simulink model "torqueBalancingPHRIStandup_2016b"  (Simulink 8.8)
settings: Solver=FixedStepDiscrete  StartTime=0.0  StopTime="Config.SIMULATION_TIME "  FixedStep=Config.Ts  RelTol=1e-3  EnableMultiTasking=on
InitFcn:
  | cd(fileparts(which(bdroot)));
  | initTorqueBalancingPHRIStandup;
StopFcn:
  | cd(fileparts(which(bdroot)));
  | stopTorqueBalancingPHRIStandup;
undefined symbols (not defined in the file or in its folder): bVectorConstraintsFeet, bVectorConstraintsLegs, Config, ConstraintsMatrixFeet, ConstraintsMatrixLegs, Gain, HUMAN_DOF_FOR_SIMULINK, Reg, ROBOT_DOF, ROBOT_DOF_FOR_SIMULINK, Sat, Sm
libraries: WBToolboxLibrary x153, simulink x4
(part 3 of 3)

== system torqueBalancingPHRIStandup_2016b/Robot system/controller_QP/Compute joint torques/QPSolver ==
  LEFT_RIGHT_FOOT_IN_CONTACT : Inport
  HessianMatrixQP1Foot : Inport  Port=2
  gradientQP1Foot : Inport  Port=3
  ConstraintsMatrixQP1Foot : Inport  Port=4
  bVectorConstraintsQP1Foot : Inport  Port=5
  HessianMatrixQP2Feet : Inport  Port=6
  gradientQP2Feet : Inport  Port=7
  ConstraintsMatrixQP2Feet : Inport  Port=8
  bVectorConstraintsQp2Feet : Inport  Port=9
  state : Inport  Port=10
  Constant1 : Constant  Value=Config.USE_QP_SOLVER
  Level-2 MATLAB S-Function : M-S-Function  FunctionName=QPBalancingStandup
  Logical Operator1 : Logic  Operator=OR  AllPortsSameDT=off  OutDataTypeStr=boolean
  ON_GAZEBO 3 : Constant  Value=Config.SCOPES_ALL
  ON_GAZEBO 4 : Constant  Value=Config.SCOPES_QP
  Visualize eventual QP failures : Subsystem
  f0OneFoot : Outport
  f0TwoFeet : Outport  Port=2
  wires:
  Level-2 MATLAB S-Function/1 -> f0TwoFeet/1
  Level-2 MATLAB S-Function/2 -> Visualize eventual QP failures/1(exitFlagQP)  "Exit flag QP two feet"
  HessianMatrixQP1Foot/1 -> Level-2 MATLAB S-Function/7
  gradientQP1Foot/1 -> Level-2 MATLAB S-Function/8
  ConstraintsMatrixQP1Foot/1 -> Level-2 MATLAB S-Function/9
  bVectorConstraintsQP1Foot/1 -> Level-2 MATLAB S-Function/10
  Level-2 MATLAB S-Function/3 -> f0OneFoot/1
  Logical Operator1/1 -> Visualize eventual QP failures/Enable
  state/1 -> Visualize eventual QP failures/2(state)
  LEFT_RIGHT_FOOT_IN_CONTACT/1 -> Level-2 MATLAB S-Function/1
  HessianMatrixQP2Feet/1 -> Level-2 MATLAB S-Function/2
  gradientQP2Feet/1 -> Level-2 MATLAB S-Function/3
  ConstraintsMatrixQP2Feet/1 -> Level-2 MATLAB S-Function/4
  bVectorConstraintsQp2Feet/1 -> Level-2 MATLAB S-Function/5
  Constant1/1 -> Level-2 MATLAB S-Function/6
  ON_GAZEBO 3/1 -> Logical Operator1/1
  ON_GAZEBO 4/1 -> Logical Operator1/2

== system torqueBalancingPHRIStandup_2016b/Human system/Dump and visualize/Human data/Using Human Model/human joint data ==
  human_jointData : Inport
  Scope : Scope  NumInputPorts=6
  head : Selector  InputPortWidth=66  IndexOptions=Index vector (dialog)  Indices=[16 17 18]  OutputSizes=1
  jointData : Scope  NumInputPorts=16
  left_ankle : Selector  InputPortWidth=66  IndexOptions=Index vector (dialog)  Indices=[61 62 63]  OutputSizes=1
  left_ball_foot : Selector  InputPortWidth=66  IndexOptions=Index vector (dialog)  Indices=[64 65 66]  OutputSizes=1
  left_elbow : Selector  InputPortWidth=66  IndexOptions=Index vector (dialog)  Indices=[37 38 39]  OutputSizes=1
  left_hip : Selector  InputPortWidth=66  IndexOptions=Index vector (dialog)  Indices=[55 56 57]  OutputSizes=1
  left_knee : Selector  InputPortWidth=66  IndexOptions=Index vector (dialog)  Indices=[58 59 60]  OutputSizes=1
  left_shoulder : Selector  InputPortWidth=66  IndexOptions=Index vector (dialog)  Indices=[34 35 36]  OutputSizes=1
  left_shoulder_internal : Selector  InputPortWidth=66  IndexOptions=Index vector (dialog)  Indices=[31 32 33]  OutputSizes=1
  left_wrist : Selector  InputPortWidth=66  IndexOptions=Index vector (dialog)  Indices=[40 41 42]  OutputSizes=1
  neck : Selector  InputPortWidth=66  IndexOptions=Index vector (dialog)  Indices=[13 14 15]  OutputSizes=1
  right_ankle : Selector  InputPortWidth=66  IndexOptions=Index vector (dialog)  Indices=[49 50 51]  OutputSizes=1
  right_ball_foot : Selector  InputPortWidth=66  IndexOptions=Index vector (dialog)  Indices=[52 53 54]  OutputSizes=1
  right_elbow : Selector  InputPortWidth=66  IndexOptions=Index vector (dialog)  Indices=[25 26 27]  OutputSizes=1
  right_hip : Selector  InputPortWidth=66  IndexOptions=Index vector (dialog)  Indices=[43 44 45]  OutputSizes=1
  right_knee : Selector  InputPortWidth=66  IndexOptions=Index vector (dialog)  Indices=[46 47 48]  OutputSizes=1
  right_shoulder : Selector  InputPortWidth=66  IndexOptions=Index vector (dialog)  Indices=[22 23 24]  OutputSizes=1
  right_shoulder_internal : Selector  InputPortWidth=66  IndexOptions=Index vector (dialog)  Indices=[19 20 21]  OutputSizes=1
  right_wrist : Selector  InputPortWidth=66  IndexOptions=Index vector (dialog)  Indices=[28 29 30]  OutputSizes=1
  torso_1 : Selector  InputPortWidth=66  IndexOptions=Index vector (dialog)  Indices=[10 11 12]  OutputSizes=1
  torso_2 : Selector  InputPortWidth=66  IndexOptions=Index vector (dialog)  Indices=[7 8 9]  OutputSizes=1
  torso_3 : Selector  InputPortWidth=66  IndexOptions=Index vector (dialog)  Indices=[4 5 6]  OutputSizes=1
  torso_4 : Selector  InputPortWidth=66  IndexOptions=Index vector (dialog)  Indices=[1 2 3]  OutputSizes=1
  wires:
  torso_1/1 -> jointData/1
  torso_4/1 -> jointData/4
  torso_3/1 -> jointData/3
  torso_2/1 -> jointData/2
  right_shoulder_internal/1 -> jointData/6
  left_shoulder_internal/1 -> jointData/5
  left_hip/1 -> jointData/7
  right_hip/1 -> jointData/8
  left_shoulder/1 -> jointData/9
  right_shoulder/1 -> jointData/10
  left_knee/1 -> jointData/11
  right_knee/1 -> jointData/12
  left_elbow/1 -> jointData/13
  right_elbow/1 -> jointData/14
  left_ankle/1 -> jointData/15
  right_ankle/1 -> jointData/16
  human_jointData/1 -> head/1, left_ball_foot/1, left_wrist/1, neck/1, right_ball_foot/1, right_wrist/1, left_shoulder/1, right_hip/1, left_hip/1, right_shoulder_internal/1, torso_1/1, torso_2/1, torso_3/1, torso_4/1, left_shoulder_internal/1, right_shoulder/1, left_knee/1, right_knee/1, left_elbow/1, right_elbow/1, right_ankle/1, left_ankle/1
  head/1 -> Scope/1
  left_ball_foot/1 -> Scope/2
  left_wrist/1 -> Scope/3
  neck/1 -> Scope/4
  right_ball_foot/1 -> Scope/5
  right_wrist/1 -> Scope/6

== system torqueBalancingPHRIStandup_2016b/Human system/Dump and visualize/Human data/Using Human Model/human joint torques data ==
  human_jointTorquesData : Inport
  Scope : Scope  NumInputPorts=6
  head : Selector  InputPortWidth=66  IndexOptions=Index vector (dialog)  Indices=[16 17 18]  OutputSizes=1
  jointTorquesData : Scope  NumInputPorts=16
  left_ankle : Selector  InputPortWidth=66  IndexOptions=Index vector (dialog)  Indices=[61 62 63]  OutputSizes=1
  left_ball_foot : Selector  InputPortWidth=66  IndexOptions=Index vector (dialog)  Indices=[64 65 66]  OutputSizes=1
  left_elbow : Selector  InputPortWidth=66  IndexOptions=Index vector (dialog)  Indices=[37 38 39]  OutputSizes=1
  left_hip : Selector  InputPortWidth=66  IndexOptions=Index vector (dialog)  Indices=[55 56 57]  OutputSizes=1
  left_knee : Selector  InputPortWidth=66  IndexOptions=Index vector (dialog)  Indices=[58 59 60]  OutputSizes=1
  left_shoulder : Selector  InputPortWidth=66  IndexOptions=Index vector (dialog)  Indices=[34 35 36]  OutputSizes=1
  left_shoulder_internal : Selector  InputPortWidth=66  IndexOptions=Index vector (dialog)  Indices=[31 32 33]  OutputSizes=1
  left_wrist : Selector  InputPortWidth=66  IndexOptions=Index vector (dialog)  Indices=[40 41 42]  OutputSizes=1
  neck : Selector  InputPortWidth=66  IndexOptions=Index vector (dialog)  Indices=[13 14 15]  OutputSizes=1
  right_ankle : Selector  InputPortWidth=66  IndexOptions=Index vector (dialog)  Indices=[49 50 51]  OutputSizes=1
  right_ball_foot : Selector  InputPortWidth=66  IndexOptions=Index vector (dialog)  Indices=[52 53 54]  OutputSizes=1
  right_elbow : Selector  InputPortWidth=66  IndexOptions=Index vector (dialog)  Indices=[25 26 27]  OutputSizes=1
  right_hip : Selector  InputPortWidth=66  IndexOptions=Index vector (dialog)  Indices=[43 44 45]  OutputSizes=1
  right_knee : Selector  InputPortWidth=66  IndexOptions=Index vector (dialog)  Indices=[46 47 48]  OutputSizes=1
  right_shoulder : Selector  InputPortWidth=66  IndexOptions=Index vector (dialog)  Indices=[22 23 24]  OutputSizes=1
  right_shoulder_internal : Selector  InputPortWidth=66  IndexOptions=Index vector (dialog)  Indices=[19 20 21]  OutputSizes=1
  right_wrist : Selector  InputPortWidth=66  IndexOptions=Index vector (dialog)  Indices=[28 29 30]  OutputSizes=1
  torso_1 : Selector  InputPortWidth=66  IndexOptions=Index vector (dialog)  Indices=[10 11 12]  OutputSizes=1
  torso_2 : Selector  InputPortWidth=66  IndexOptions=Index vector (dialog)  Indices=[7 8 9]  OutputSizes=1
  torso_3 : Selector  InputPortWidth=66  IndexOptions=Index vector (dialog)  Indices=[4 5 6]  OutputSizes=1
  torso_4 : Selector  InputPortWidth=66  IndexOptions=Index vector (dialog)  Indices=[1 2 3]  OutputSizes=1
  wires:
  torso_1/1 -> jointTorquesData/1
  torso_4/1 -> jointTorquesData/4
  torso_3/1 -> jointTorquesData/3
  torso_2/1 -> jointTorquesData/2
  right_shoulder_internal/1 -> jointTorquesData/6
  left_shoulder_internal/1 -> jointTorquesData/5
  left_hip/1 -> jointTorquesData/7
  right_hip/1 -> jointTorquesData/8
  left_shoulder/1 -> jointTorquesData/9
  right_shoulder/1 -> jointTorquesData/10
  left_knee/1 -> jointTorquesData/11
  right_knee/1 -> jointTorquesData/12
  left_elbow/1 -> jointTorquesData/13
  right_elbow/1 -> jointTorquesData/14
  left_ankle/1 -> jointTorquesData/15
  right_ankle/1 -> jointTorquesData/16
  human_jointTorquesData/1 -> head/1, left_ball_foot/1, left_wrist/1, neck/1, right_ball_foot/1, right_wrist/1, left_shoulder/1, right_hip/1, left_hip/1, right_shoulder_internal/1, torso_1/1, torso_2/1, torso_3/1, torso_4/1, left_shoulder_internal/1, right_shoulder/1, left_knee/1, right_knee/1, left_elbow/1, right_elbow/1, right_ankle/1, left_ankle/1
  head/1 -> Scope/1
  left_ball_foot/1 -> Scope/2
  left_wrist/1 -> Scope/3
  neck/1 -> Scope/4
  right_ball_foot/1 -> Scope/5
  right_wrist/1 -> Scope/6

== system torqueBalancingPHRIStandup_2016b/Human system/Dump and visualize/Human data/Using Human Model/human joint velocities data ==
  human_jointVelocitiesData : Inport
  Scope : Scope  NumInputPorts=6
  head : Selector  InputPortWidth=66  IndexOptions=Index vector (dialog)  Indices=[16 17 18]  OutputSizes=1
  jointVelocitiesData : Scope  NumInputPorts=16
  left_ankle : Selector  InputPortWidth=66  IndexOptions=Index vector (dialog)  Indices=[61 62 63]  OutputSizes=1
  left_ball_foot : Selector  InputPortWidth=66  IndexOptions=Index vector (dialog)  Indices=[64 65 66]  OutputSizes=1
  left_elbow : Selector  InputPortWidth=66  IndexOptions=Index vector (dialog)  Indices=[37 38 39]  OutputSizes=1
  left_hip : Selector  InputPortWidth=66  IndexOptions=Index vector (dialog)  Indices=[55 56 57]  OutputSizes=1
  left_knee : Selector  InputPortWidth=66  IndexOptions=Index vector (dialog)  Indices=[58 59 60]  OutputSizes=1
  left_shoulder : Selector  InputPortWidth=66  IndexOptions=Index vector (dialog)  Indices=[34 35 36]  OutputSizes=1
  left_shoulder_internal : Selector  InputPortWidth=66  IndexOptions=Index vector (dialog)  Indices=[31 32 33]  OutputSizes=1
  left_wrist : Selector  InputPortWidth=66  IndexOptions=Index vector (dialog)  Indices=[40 41 42]  OutputSizes=1
  neck : Selector  InputPortWidth=66  IndexOptions=Index vector (dialog)  Indices=[13 14 15]  OutputSizes=1
  right_ankle : Selector  InputPortWidth=66  IndexOptions=Index vector (dialog)  Indices=[49 50 51]  OutputSizes=1
  right_ball_foot : Selector  InputPortWidth=66  IndexOptions=Index vector (dialog)  Indices=[52 53 54]  OutputSizes=1
  right_elbow : Selector  InputPortWidth=66  IndexOptions=Index vector (dialog)  Indices=[25 26 27]  OutputSizes=1
  right_hip : Selector  InputPortWidth=66  IndexOptions=Index vector (dialog)  Indices=[43 44 45]  OutputSizes=1
  right_knee : Selector  InputPortWidth=66  IndexOptions=Index vector (dialog)  Indices=[46 47 48]  OutputSizes=1
  right_shoulder : Selector  InputPortWidth=66  IndexOptions=Index vector (dialog)  Indices=[22 23 24]  OutputSizes=1
  right_shoulder_internal : Selector  InputPortWidth=66  IndexOptions=Index vector (dialog)  Indices=[19 20 21]  OutputSizes=1
  right_wrist : Selector  InputPortWidth=66  IndexOptions=Index vector (dialog)  Indices=[28 29 30]  OutputSizes=1
  torso_1 : Selector  InputPortWidth=66  IndexOptions=Index vector (dialog)  Indices=[10 11 12]  OutputSizes=1
  torso_2 : Selector  InputPortWidth=66  IndexOptions=Index vector (dialog)  Indices=[7 8 9]  OutputSizes=1
  torso_3 : Selector  InputPortWidth=66  IndexOptions=Index vector (dialog)  Indices=[4 5 6]  OutputSizes=1
  torso_4 : Selector  InputPortWidth=66  IndexOptions=Index vector (dialog)  Indices=[1 2 3]  OutputSizes=1
  wires:
  torso_1/1 -> jointVelocitiesData/1
  torso_4/1 -> jointVelocitiesData/4
  torso_3/1 -> jointVelocitiesData/3
  torso_2/1 -> jointVelocitiesData/2
  right_shoulder_internal/1 -> jointVelocitiesData/6
  left_shoulder_internal/1 -> jointVelocitiesData/5
  left_hip/1 -> jointVelocitiesData/7
  right_hip/1 -> jointVelocitiesData/8
  left_shoulder/1 -> jointVelocitiesData/9
  right_shoulder/1 -> jointVelocitiesData/10
  left_knee/1 -> jointVelocitiesData/11
  right_knee/1 -> jointVelocitiesData/12
  left_elbow/1 -> jointVelocitiesData/13
  right_elbow/1 -> jointVelocitiesData/14
  left_ankle/1 -> jointVelocitiesData/15
  right_ankle/1 -> jointVelocitiesData/16
  human_jointVelocitiesData/1 -> head/1, left_ball_foot/1, left_wrist/1, neck/1, right_ball_foot/1, right_wrist/1, left_shoulder/1, right_hip/1, left_hip/1, right_shoulder_internal/1, torso_1/1, torso_2/1, torso_3/1, torso_4/1, left_shoulder_internal/1, right_shoulder/1, left_knee/1, right_knee/1, left_elbow/1, right_elbow/1, right_ankle/1, left_ankle/1
  head/1 -> Scope/1
  left_ball_foot/1 -> Scope/2
  left_wrist/1 -> Scope/3
  neck/1 -> Scope/4
  right_ball_foot/1 -> Scope/5
  right_wrist/1 -> Scope/6

== system torqueBalancingPHRIStandup_2016b/Robot system/Robot State and References/Internal Coordinator/Base to fixed_link/LFoot to base link transform  ==
  qj : Inport
  inertial : Inport  Port=2
  w_H_link : Inport  Port=3
  w_H_base_fixed : Inport  Port=4
  Fixed base to imu transform : WBToolboxLibrary/wholeBodyModel/Kinematics/Forward Kinematics  frameName=Frames.IMU
  Fixed base to root link transform : WBToolboxLibrary/wholeBodyModel/Kinematics/Forward Kinematics  frameName=Frames.BASE
  Inv\* : Product  Inputs=/*  Multiplication=Matrix(*)
  "Inv\\*  " : Product  Inputs=/*  Multiplication=Matrix(*)
  Neck Position : WBToolboxLibrary/Utilities/Yarp Read  portName=Ports.NECK_POS  signalSize=6  timeout=0.5  blocking=off  timestamp=off  autoconnect=on  errorOnConnection=off
  Switch6 : Switch  Criteria=u2 > Threshold
  USE_IMU4EST_BASE : Constant  Value=Config.USE_IMU4EST_BASE
  fromImuToHomogeousTransformFCN : MATLAB Function  TreatAsAtomicUnit=on
  holder 1 : WBToolboxLibrary/Utilities/holder 
  holder 2 : WBToolboxLibrary/Utilities/holder 
  neck transform : Subsystem
  link_H_b : Outport
  wires:
  Switch6/1 -> link_H_b/1
  "Inv\\*  "/1 -> Switch6/3, fromImuToHomogeousTransformFCN/3(link_H_base)  "link_H_root"
  USE_IMU4EST_BASE/1 -> Switch6/2
  Inv\*/1 -> fromImuToHomogeousTransformFCN/1(imu_H_link), holder 1/1  "imu_H_link"
  holder 2/1 -> fromImuToHomogeousTransformFCN/4(inertial_0)
  Fixed base to imu transform/1 -> Inv\*/1
  holder 1/1 -> fromImuToHomogeousTransformFCN/2(imu_H_link_0)
  qj/1 -> Fixed base to imu transform/2, Fixed base to root link transform/2
  fromImuToHomogeousTransformFCN/1(w_H_b) -> Switch6/1
  Fixed base to root link transform/1 -> "Inv\\*  "/2
  inertial/1 -> holder 2/1, fromImuToHomogeousTransformFCN/5(inertial)
  Neck Position/1 -> neck transform/1(neck port)
  neck transform/1(neck position) -> fromImuToHomogeousTransformFCN/6(neck_pos)
  w_H_link/1 -> "Inv\\*  "/1, Inv\*/2
  w_H_base_fixed/1 -> Fixed base to root link transform/1, Fixed base to imu transform/1

== system torqueBalancingPHRIStandup_2016b/Robot system/Robot State and References/Internal Coordinator/Compute State Velocity/Feet Jacobians ==
  qj : Inport
  w_H_b : Inport  Port=2
  Jacobian LFoot : WBToolboxLibrary/wholeBodyModel/Jacobians/Jacobian  frameName=Frames.LEFT_FOOT
  Jacobian RFoot : WBToolboxLibrary/wholeBodyModel/Jacobians/Jacobian  frameName=Frames.RIGHT_FOOT
  J_LFoot : Outport
  J_RFoot : Outport  Port=2
  wires:
  Jacobian LFoot/1 -> J_LFoot/1
  Jacobian RFoot/1 -> J_RFoot/1
  w_H_b/1 -> Jacobian RFoot/1, Jacobian LFoot/1
  qj/1 -> Jacobian LFoot/2, Jacobian RFoot/2

== system torqueBalancingPHRIStandup_2016b/Robot system/Robot State and References/State Machine Standup/Compute State Velocity/Fixed Links Jacobians ==
  "state " : Inport
  qj : Inport  Port=2
  w_H_b : Inport  Port=3
  " " : WBToolboxLibrary/wholeBodyModel/Jacobians/Jacobian  frameName=Frames.LEFT_LEG
  "  " : WBToolboxLibrary/wholeBodyModel/Jacobians/Jacobian  frameName=Frames.RIGHT_LEG
  "   " : WBToolboxLibrary/wholeBodyModel/Jacobians/Jacobian  frameName=Frames.RIGHT_FOOT
  "       " : WBToolboxLibrary/wholeBodyModel/Jacobians/Jacobian  frameName=Frames.LEFT_FOOT
  Constant : Constant  Value=Config.iCubStandUp
  Legs in Contact : MATLAB Function  TreatAsAtomicUnit=on
  Switch1 : Switch  Criteria=u2 > Threshold  Threshold=0.1
  Switch2 : Switch  Criteria=u2 > Threshold  Threshold=0.1
  J_LeftFixed : Outport
  J_RightFixed : Outport  Port=2
  wires:
  Switch2/1 -> J_RightFixed/1
  Legs in Contact/1(legsInContact) -> Switch2/2, Switch1/2
  " "/1 -> Switch1/1
  "       "/1 -> Switch1/3
  "   "/1 -> Switch2/3
  "  "/1 -> Switch2/1
  "state "/1 -> Legs in Contact/2(state)
  Constant/1 -> Legs in Contact/1(icubStandup)
  Switch1/1 -> J_LeftFixed/1
  qj/1 -> "   "/2, "  "/2, "       "/2, " "/2
  w_H_b/1 -> "   "/1, " "/1, "       "/1, "  "/1

== system torqueBalancingPHRIStandup_2016b/Robot system/Robot State and References/State Machine Standup/Compute base to fixed link transform/LFoot to base link transform  ==
  qj : Inport
  inertial : Inport  Port=2
  w_H_link : Inport  Port=3
  w_H_base_fixed : Inport  Port=4
  Fixed base to imu transform : WBToolboxLibrary/wholeBodyModel/Kinematics/Forward Kinematics  frameName=Frames.IMU
  Fixed base to root link transform : WBToolboxLibrary/wholeBodyModel/Kinematics/Forward Kinematics  frameName=Frames.BASE
  Inv\* : Product  Inputs=/*  Multiplication=Matrix(*)
  "Inv\\*  " : Product  Inputs=/*  Multiplication=Matrix(*)
  Neck Position : WBToolboxLibrary/Utilities/Yarp Read  portName=Ports.NECK_POS  signalSize=6  timeout=0.5  blocking=off  timestamp=off  autoconnect=on  errorOnConnection=off
  Switch6 : Switch  Criteria=u2 > Threshold
  USE_IMU4EST_BASE : Constant  Value=Config.USE_IMU4EST_BASE
  fromImuToHomogeousTransformFCN : MATLAB Function  TreatAsAtomicUnit=on
  holder 1 : WBToolboxLibrary/Utilities/holder 
  holder 2 : WBToolboxLibrary/Utilities/holder 
  neck transform : Subsystem
  link_H_b : Outport
  wires:
  Switch6/1 -> link_H_b/1
  "Inv\\*  "/1 -> Switch6/3, fromImuToHomogeousTransformFCN/3(link_H_base)  "link_H_root"
  USE_IMU4EST_BASE/1 -> Switch6/2
  Inv\*/1 -> fromImuToHomogeousTransformFCN/1(imu_H_link), holder 1/1  "imu_H_link"
  holder 2/1 -> fromImuToHomogeousTransformFCN/4(inertial_0)
  Fixed base to imu transform/1 -> Inv\*/1
  holder 1/1 -> fromImuToHomogeousTransformFCN/2(imu_H_link_0)
  qj/1 -> Fixed base to imu transform/2, Fixed base to root link transform/2
  fromImuToHomogeousTransformFCN/1(w_H_b) -> Switch6/1
  Fixed base to root link transform/1 -> "Inv\\*  "/2
  inertial/1 -> holder 2/1, fromImuToHomogeousTransformFCN/5(inertial)
  Neck Position/1 -> neck transform/1(neck port)
  neck transform/1(neck position) -> fromImuToHomogeousTransformFCN/6(neck_pos)
  w_H_link/1 -> "Inv\\*  "/1, Inv\*/2
  w_H_base_fixed/1 -> Fixed base to root link transform/1, Fixed base to imu transform/1

== system torqueBalancingPHRIStandup_2016b/Robot system/Robot State and References/State Machine Standup/Compute base to fixed link transform/LLeg to base link transform ==
  qj : Inport
  inertial : Inport  Port=2
  w_H_link : Inport  Port=3
  w_H_base_fixed : Inport  Port=4
  Fixed base to imu transform : WBToolboxLibrary/wholeBodyModel/Kinematics/Forward Kinematics  frameName=Frames.IMU
  Fixed base to root link transform : WBToolboxLibrary/wholeBodyModel/Kinematics/Forward Kinematics  frameName=Frames.BASE
  Inv\* : Product  Inputs=/*  Multiplication=Matrix(*)
  "Inv\\*  " : Product  Inputs=/*  Multiplication=Matrix(*)
  Neck Position : WBToolboxLibrary/Utilities/Yarp Read  portName=Ports.NECK_POS  signalSize=6  timeout=0.5  blocking=off  timestamp=off  autoconnect=on  errorOnConnection=off
  Switch6 : Switch  Criteria=u2 > Threshold
  USE_IMU4EST_BASE : Constant  Value=Config.USE_IMU4EST_BASE
  fromImuToHomogeousTransformFCN : MATLAB Function  TreatAsAtomicUnit=on
  holder 1 : WBToolboxLibrary/Utilities/holder 
  holder 2 : WBToolboxLibrary/Utilities/holder 
  neck transform : Subsystem
  link_H_b : Outport
  wires:
  Switch6/1 -> link_H_b/1
  "Inv\\*  "/1 -> Switch6/3, fromImuToHomogeousTransformFCN/3(link_H_base)  "link_H_root"
  USE_IMU4EST_BASE/1 -> Switch6/2
  Inv\*/1 -> fromImuToHomogeousTransformFCN/1(imu_H_link), holder 1/1  "imu_H_link"
  holder 2/1 -> fromImuToHomogeousTransformFCN/4(inertial_0)
  Fixed base to imu transform/1 -> Inv\*/1
  holder 1/1 -> fromImuToHomogeousTransformFCN/2(imu_H_link_0)
  qj/1 -> Fixed base to imu transform/2, Fixed base to root link transform/2
  fromImuToHomogeousTransformFCN/1(w_H_b) -> Switch6/1
  Fixed base to root link transform/1 -> "Inv\\*  "/2
  inertial/1 -> holder 2/1, fromImuToHomogeousTransformFCN/5(inertial)
  Neck Position/1 -> neck transform/1(neck port)
  neck transform/1(neck position) -> fromImuToHomogeousTransformFCN/6(neck_pos)
  w_H_link/1 -> "Inv\\*  "/1, Inv\*/2
  w_H_base_fixed/1 -> Fixed base to root link transform/1, Fixed base to imu transform/1

== system torqueBalancingPHRIStandup_2016b/Robot system/controller_QP/Compute angular momentum integral/Compute base to fixed link transform/LFoot to base link transform  ==
  qj : Inport
  inertial : Inport  Port=2
  w_H_link : Inport  Port=3
  w_H_base_fixed : Inport  Port=4
  Fixed base to imu transform : WBToolboxLibrary/wholeBodyModel/Kinematics/Forward Kinematics  frameName=Frames.IMU
  Fixed base to root link transform : WBToolboxLibrary/wholeBodyModel/Kinematics/Forward Kinematics  frameName=Frames.BASE
  Inv\* : Product  Inputs=/*  Multiplication=Matrix(*)
  "Inv\\*  " : Product  Inputs=/*  Multiplication=Matrix(*)
  Neck Position : WBToolboxLibrary/Utilities/Yarp Read  portName=Ports.NECK_POS  signalSize=6  timeout=0.5  blocking=off  timestamp=off  autoconnect=on  errorOnConnection=off
  Switch6 : Switch  Criteria=u2 > Threshold
  USE_IMU4EST_BASE : Constant  Value=Config.USE_IMU4EST_BASE
  fromImuToHomogeousTransformFCN : MATLAB Function  TreatAsAtomicUnit=on
  holder 1 : WBToolboxLibrary/Utilities/holder 
  holder 2 : WBToolboxLibrary/Utilities/holder 
  neck transform : Subsystem
  link_H_b : Outport
  wires:
  Switch6/1 -> link_H_b/1
  "Inv\\*  "/1 -> Switch6/3, fromImuToHomogeousTransformFCN/3(link_H_base)  "link_H_root"
  USE_IMU4EST_BASE/1 -> Switch6/2
  Inv\*/1 -> fromImuToHomogeousTransformFCN/1(imu_H_link), holder 1/1  "imu_H_link"
  holder 2/1 -> fromImuToHomogeousTransformFCN/4(inertial_0)
  Fixed base to imu transform/1 -> Inv\*/1
  holder 1/1 -> fromImuToHomogeousTransformFCN/2(imu_H_link_0)
  qj/1 -> Fixed base to imu transform/2, Fixed base to root link transform/2
  fromImuToHomogeousTransformFCN/1(w_H_b) -> Switch6/1
  Fixed base to root link transform/1 -> "Inv\\*  "/2
  inertial/1 -> holder 2/1, fromImuToHomogeousTransformFCN/5(inertial)
  Neck Position/1 -> neck transform/1(neck port)
  neck transform/1(neck position) -> fromImuToHomogeousTransformFCN/6(neck_pos)
  w_H_link/1 -> "Inv\\*  "/1, Inv\*/2
  w_H_base_fixed/1 -> Fixed base to root link transform/1, Fixed base to imu transform/1

== system torqueBalancingPHRIStandup_2016b/Robot system/controller_QP/Compute angular momentum integral/Compute base to fixed link transform/LLeg to base link transform ==
  qj : Inport
  inertial : Inport  Port=2
  w_H_link : Inport  Port=3
  w_H_base_fixed : Inport  Port=4
  Fixed base to imu transform : WBToolboxLibrary/wholeBodyModel/Kinematics/Forward Kinematics  frameName=Frames.IMU
  Fixed base to root link transform : WBToolboxLibrary/wholeBodyModel/Kinematics/Forward Kinematics  frameName=Frames.BASE
  Inv\* : Product  Inputs=/*  Multiplication=Matrix(*)
  "Inv\\*  " : Product  Inputs=/*  Multiplication=Matrix(*)
  Neck Position : WBToolboxLibrary/Utilities/Yarp Read  portName=Ports.NECK_POS  signalSize=6  timeout=0.5  blocking=off  timestamp=off  autoconnect=on  errorOnConnection=off
  Switch6 : Switch  Criteria=u2 > Threshold
  USE_IMU4EST_BASE : Constant  Value=Config.USE_IMU4EST_BASE
  fromImuToHomogeousTransformFCN : MATLAB Function  TreatAsAtomicUnit=on
  holder 1 : WBToolboxLibrary/Utilities/holder 
  holder 2 : WBToolboxLibrary/Utilities/holder 
  neck transform : Subsystem
  link_H_b : Outport
  wires:
  Switch6/1 -> link_H_b/1
  "Inv\\*  "/1 -> Switch6/3, fromImuToHomogeousTransformFCN/3(link_H_base)  "link_H_root"
  USE_IMU4EST_BASE/1 -> Switch6/2
  Inv\*/1 -> fromImuToHomogeousTransformFCN/1(imu_H_link), holder 1/1  "imu_H_link"
  holder 2/1 -> fromImuToHomogeousTransformFCN/4(inertial_0)
  Fixed base to imu transform/1 -> Inv\*/1
  holder 1/1 -> fromImuToHomogeousTransformFCN/2(imu_H_link_0)
  qj/1 -> Fixed base to imu transform/2, Fixed base to root link transform/2
  fromImuToHomogeousTransformFCN/1(w_H_b) -> Switch6/1
  Fixed base to root link transform/1 -> "Inv\\*  "/2
  inertial/1 -> holder 2/1, fromImuToHomogeousTransformFCN/5(inertial)
  Neck Position/1 -> neck transform/1(neck port)
  neck transform/1(neck position) -> fromImuToHomogeousTransformFCN/6(neck_pos)
  w_H_link/1 -> "Inv\\*  "/1, Inv\*/2
  w_H_base_fixed/1 -> Fixed base to root link transform/1, Fixed base to imu transform/1

== system torqueBalancingPHRIStandup_2016b/Robot system/controller_QP/Compute joint torques/QPSolver/Visualize eventual QP failures ==
  exitFlagQP : Inport
  state : Inport  Port=2
  Enable : EnablePort
  "QP status (0: no failure, 1: not using)" : Scope  NumInputPorts=2
  wires:
  exitFlagQP/1 -> "QP status (0: no failure, 1: not using)"/1  "exitFlagQP"
  state/1 -> "QP status (0: no failure, 1: not using)"/2

== system torqueBalancingPHRIStandup_2016b/Robot system/Robot State and References/Internal Coordinator/Base to fixed_link/LFoot to base link transform /neck transform ==
  neck port : Inport
  Constant : Constant  Value=zeros(3,1)
  Gain : Gain  Gain=pi/180
  Selector1 : Selector  InputPortWidth=6  IndexOptions=Index vector (dialog)  Indices=[1:3]  OutputSizes=1
  Switch : Switch  Criteria=u2 > Threshold
  USE_IMU4EST_BASE1 : Constant  Value=Config.CORRECT_NECK_IMU
  neck position : Outport
  wires:
  neck port/1 -> Gain/1
  USE_IMU4EST_BASE1/1 -> Switch/2
  Switch/1 -> neck position/1
  Gain/1 -> Selector1/1
  Constant/1 -> Switch/3
  Selector1/1 -> Switch/1  "neck pos"

== system torqueBalancingPHRIStandup_2016b/Robot system/Robot State and References/State Machine Standup/Compute base to fixed link transform/LFoot to base link transform /neck transform ==
  neck port : Inport
  Constant : Constant  Value=zeros(3,1)
  Gain : Gain  Gain=pi/180
  Selector1 : Selector  InputPortWidth=6  IndexOptions=Index vector (dialog)  Indices=[1:3]  OutputSizes=1
  Switch : Switch  Criteria=u2 > Threshold
  USE_IMU4EST_BASE1 : Constant  Value=Config.CORRECT_NECK_IMU
  neck position : Outport
  wires:
  neck port/1 -> Gain/1
  USE_IMU4EST_BASE1/1 -> Switch/2
  Switch/1 -> neck position/1
  Gain/1 -> Selector1/1
  Constant/1 -> Switch/3
  Selector1/1 -> Switch/1  "neck pos"

== system torqueBalancingPHRIStandup_2016b/Robot system/Robot State and References/State Machine Standup/Compute base to fixed link transform/LLeg to base link transform/neck transform ==
  neck port : Inport
  Constant : Constant  Value=zeros(3,1)
  Gain : Gain  Gain=pi/180
  Selector1 : Selector  InputPortWidth=6  IndexOptions=Index vector (dialog)  Indices=[1:3]  OutputSizes=1
  Switch : Switch  Criteria=u2 > Threshold
  USE_IMU4EST_BASE1 : Constant  Value=Config.CORRECT_NECK_IMU
  neck position : Outport
  wires:
  neck port/1 -> Gain/1
  USE_IMU4EST_BASE1/1 -> Switch/2
  Switch/1 -> neck position/1
  Gain/1 -> Selector1/1
  Constant/1 -> Switch/3
  Selector1/1 -> Switch/1  "neck pos"

== system torqueBalancingPHRIStandup_2016b/Robot system/controller_QP/Compute angular momentum integral/Compute base to fixed link transform/LFoot to base link transform /neck transform ==
  neck port : Inport
  Constant : Constant  Value=zeros(3,1)
  Gain : Gain  Gain=pi/180
  Selector1 : Selector  InputPortWidth=6  IndexOptions=Index vector (dialog)  Indices=[1:3]  OutputSizes=1
  Switch : Switch  Criteria=u2 > Threshold
  USE_IMU4EST_BASE1 : Constant  Value=Config.CORRECT_NECK_IMU
  neck position : Outport
  wires:
  neck port/1 -> Gain/1
  USE_IMU4EST_BASE1/1 -> Switch/2
  Switch/1 -> neck position/1
  Gain/1 -> Selector1/1
  Constant/1 -> Switch/3
  Selector1/1 -> Switch/1  "neck pos"

== system torqueBalancingPHRIStandup_2016b/Robot system/controller_QP/Compute angular momentum integral/Compute base to fixed link transform/LLeg to base link transform/neck transform ==
  neck port : Inport
  Constant : Constant  Value=zeros(3,1)
  Gain : Gain  Gain=pi/180
  Selector1 : Selector  InputPortWidth=6  IndexOptions=Index vector (dialog)  Indices=[1:3]  OutputSizes=1
  Switch : Switch  Criteria=u2 > Threshold
  USE_IMU4EST_BASE1 : Constant  Value=Config.CORRECT_NECK_IMU
  neck position : Outport
  wires:
  neck port/1 -> Gain/1
  USE_IMU4EST_BASE1/1 -> Switch/2
  Switch/1 -> neck position/1
  Gain/1 -> Selector1/1
  Constant/1 -> Switch/3
  Selector1/1 -> Switch/1  "neck pos"

== matlab function Robot system/controller_QP/Compute angular momentum integral/Compute base to fixed link transform/LFoot to base link transform /fromImuToHomogeousTransformFCN ==
  data: imu_H_link input double; imu_H_link_0 input double; link_H_base input double; inertial_0 input double; inertial input double; neck_pos input double; w_H_b output double; Config parameter double
function w_H_b = worldToBaseTransformWithIMUFCN(imu_H_link,imu_H_link_0,link_H_base,inertial_0,inertial,neck_pos,Config)

    w_H_b = worldToBaseTransformWithIMU(imu_H_link,imu_H_link_0,link_H_base,inertial_0,inertial,neck_pos,Config);

end

== matlab function Robot system/Robot State and References/Internal Coordinator/Base to fixed_link/LFoot to base link transform /fromImuToHomogeousTransformFCN ==
  data: imu_H_link input double; imu_H_link_0 input double; link_H_base input double; inertial_0 input double; inertial input double; neck_pos input double; w_H_b output double; Config parameter double
function w_H_b = worldToBaseTransformWithIMUFCN(imu_H_link,imu_H_link_0,link_H_base,inertial_0,inertial,neck_pos,Config)

    w_H_b = worldToBaseTransformWithIMU(imu_H_link,imu_H_link_0,link_H_base,inertial_0,inertial,neck_pos,Config);

end

== matlab function Robot system/Robot State and References/State Machine Standup/Compute base to fixed link transform/LLeg to base link transform/fromImuToHomogeousTransformFCN ==
  data: imu_H_link input double; imu_H_link_0 input double; link_H_base input double; inertial_0 input double; inertial input double; neck_pos input double; w_H_b output double; Config parameter double
function w_H_b = worldToBaseTransformWithIMUFCN(imu_H_link,imu_H_link_0,link_H_base,inertial_0,inertial,neck_pos,Config)

    w_H_b = worldToBaseTransformWithIMU(imu_H_link,imu_H_link_0,link_H_base,inertial_0,inertial,neck_pos,Config);

end

== matlab function Robot system/controller_QP/Compute angular momentum integral/Compute base to fixed link transform/LLeg to base link transform/fromImuToHomogeousTransformFCN ==
  data: imu_H_link input double; imu_H_link_0 input double; link_H_base input double; inertial_0 input double; inertial input double; neck_pos input double; w_H_b output double; Config parameter double
function w_H_b = worldToBaseTransformWithIMUFCN(imu_H_link,imu_H_link_0,link_H_base,inertial_0,inertial,neck_pos,Config)

    w_H_b = worldToBaseTransformWithIMU(imu_H_link,imu_H_link_0,link_H_base,inertial_0,inertial,neck_pos,Config);

end

== matlab function Robot system/Robot State and References/Internal Coordinator/Compute State Velocity/Compute Base Velocity ==
  data: J_LeftFoot input double; J_RightFoot input double; feetInContact input double; nu_b output double; qjDot input double; Reg parameter double
function nu_b = computeBaseVelocityFCN(J_LeftFoot, J_RightFoot, feetInContact, qjDot, Reg)

    nu_b = computeBaseVelocity(J_LeftFoot, J_RightFoot, feetInContact, qjDot, Reg);
end

== matlab function Robot system/Dynamics and Kinematics/Dynamics/Add motors reflected inertias/Add motor reflected inertias ==
  data: M input double; M_with_inertia output double; Config parameter double
function M_with_inertia = addMotorsInertiaFCN(M,Config)

    M_with_inertia = addMotorsInertia(M,Config);

end

== matlab function Robot system/Robot State and References/State Machine Standup/Compute State Velocity/Compute Base Velocity ==
  data: J_LeftFixedLink input double; J_RightFixedLink input double; feetInContact input double; nu_b output double; qjDot input double; Reg parameter double
function nu_b = computeBaseVelocityFCN(J_LeftFixedLink, J_RightFixedLink, feetInContact, qjDot, Reg)

    nu_b = computeBaseVelocity(J_LeftFixedLink, J_RightFixedLink, feetInContact, qjDot, Reg);
end

== matlab function Robot system/Robot State and References/State Machine Standup/Compute base to fixed link transform/LFoot to base link transform /fromImuToHomogeousTransformFCN ==
  data: imu_H_link input double; imu_H_link_0 input double; link_H_base input double; inertial_0 input double; inertial input double; neck_pos input double; w_H_b output double; Config parameter double
function w_H_b = worldToBaseTransformWithIMUFCN(imu_H_link,imu_H_link_0,link_H_base,inertial_0,inertial,neck_pos,Config)

    w_H_b = worldToBaseTransformWithIMU(imu_H_link,imu_H_link_0,link_H_base,inertial_0,inertial,neck_pos,Config);

end

== matlab function Robot system/Dynamics and Kinematics/Kinematics/Legs in Contact ==
  data: icubStandup input double; legsInContact output double; state input double
function legsInContact = legsContactDetectorFCN(icubStandup,state)

   legsInContact = legsContactDetector(icubStandup,state);
end

== matlab function Robot system/Robot State and References/Internal Coordinator/Reference Generator CoM ==
  data: pos_CoM_0 input double; t input double; references_CoM output double; Config parameter double
function references_CoM = referenceGeneratorCoMFCN(pos_CoM_0, t, Config)

    references_CoM = referenceGeneratorCoM(pos_CoM_0, t, Config);
end

== matlab function Robot system/controller_QP/Compute angular momentum integral/Legs in Contact ==
  data: icubStandup input double; legsInContact output double; state input double
function legsInContact = legsContactDetectorFCN(icubStandup,state)

   legsInContact = legsContactDetector(icubStandup,state);
end

== matlab function Robot system/controller_QP/Compute joint torques (motor reflected inertia)/(transpose(T*Gamma))^{-1}*I_m*(T*Gamma)^{-1} ==
  data: reflectedInertia output double; Config parameter double
function reflectedInertia  = computeMotorsInertiaFCN(Config)

    [reflectedInertia] = computeMotorsInertia(Config);

end

== matlab function Robot system/Robot State and References/State Machine Standup/stateMachineStandupFCN ==
  data: wrench_rightFoot input double; wrench_leftFoot input double; w_H_b output double; constraints output double; CoM_des output double; qj_des output double; wrench_leftHand input double; wrench_rightHand input double; xCoM_0 input double; qj_0 input double; xCoM input double; l_sole_H_b input double; l_upper_leg_contact_H_b input double; t input double; STANDUP_WITH_HUMAN_FORCE input double; MEASURED_FT input double; STANDUP_WITH_HUMAN_TORQUE input double; Sm parameter double; impedances output double; KPCoM output double; KDCoM output double; Gain parameter double; currentState output double; jointsAndCoMSmoothingTime output double; fArms_phri input double
function [w_H_b, constraints, CoM_des, qj_des, impedances, KPCoM, KDCoM, currentState, jointsAndCoMSmoothingTime] = ...
             stateMachineStandupFCN(wrench_rightFoot, wrench_leftFoot, wrench_leftHand, wrench_rightHand, xCoM_0, qj_0, xCoM, l_sole_H_b, l_upper_leg_contact_H_b, t, STANDUP_WITH_HUMAN_FORCE, MEASURED_FT, STANDUP_WITH_HUMAN_TORQUE, Sm, Gain, fArms_phri)
         
         [w_H_b, constraints, CoM_des, qj_des, impedances, KPCoM, KDCoM, currentState, jointsAndCoMSmoothingTime] = ...
             stateMachineStandup(wrench_rightFoot, wrench_leftFoot, wrench_leftHand, wrench_rightHand, xCoM_0, qj_0, xCoM, l_sole_H_b, l_upper_leg_contact_H_b, t, STANDUP_WITH_HUMAN_FORCE, MEASURED_FT, STANDUP_WITH_HUMAN_TORQUE, Sm, Gain, fArms_phri);
end

== matlab function Robot system/Robot State and References/State Machine Standup/Compute State Velocity/Fixed Links Jacobians/Legs in Contact ==
  data: icubStandup input double; legsInContact output double; state input double
function legsInContact = legsContactDetectorFCN(icubStandup,state)

   legsInContact = legsContactDetector(icubStandup,state);
end

== matlab function Robot system/robot world to human feet transformation/MATLAB Function ==
  data: w_H_humanLeftFeet output double; w_H_robotLeftFeet input double; w_H_robotRightFeet input double; w_H_humanRightFeet output double
function [w_H_humanLeftFeet, w_H_humanRightFeet ]= fcn(w_H_robotLeftFeet,w_H_robotRightFeet)

    %% Fixed transformation from the robot feet to human feet defined
    %  human-forces-provider module configuration
    robotLeftFeet_H_humanLeftFeet = [-1.0   0.0     0.0     0.59;
                                      0.0  -1.0     0.0    -0.2549;
                                      0.0   0.0     1.0     0.0;
                                      0.0   0.0     0.0     1.0];
                                  
    robotRightFeet_H_humanRightFeet = [-1.0   0.0     0.0     0.59;
                                        0.0  -1.0     0.0    -0.2549;
                                        0.0   0.0     1.0     0.0;
                                        0.0   0.0     0.0     1.0];
                                  
    w_H_humanLeftFeet  = w_H_robotLeftFeet * robotLeftFeet_H_humanLeftFeet;
    
    w_H_humanRightFeet = w_H_robotRightFeet * robotRightFeet_H_humanRightFeet;

end

== matlab function Human system/Robot Model Position Control/getJointRef ==
  data: sim_time input double; q input double; state input double; joint_ref output double
function joint_ref = getJointRef(sim_time, q, state)

    joint_ref        = q;
    joint_references = [-0.2973   -0.0000   -0.0000   -0.1376    0.1919   -0.0000    0.5629   -0.1376    0.1929   -0.0000    0.5629   -0.0003   -0.0001   -0.0001   -0.0008    0.0012    0.0001   -0.0004    0.0000    0.0001   -0.0008    0.0012   -0.0001;
                         0.1873    0.0000   -0.0000    0.1296    0.1901    0.0019    0.6084    0.1296    0.1901    0.0019    0.6084   -0.0007   -0.0001   -0.0001   -0.0017    0.0025    0.0001   -0.0007   -0.0000    0.0000   -0.0017    0.0025   -0.0001;
                         0.1873   -0.0000   -0.0000    0.1217    0.1896   -0.0004    1.1403    0.1217    0.1896   -0.0004    1.1403   -0.0014   -0.0001   -0.0000   -0.0023    0.0032    0.0000   -0.0014   -0.0000    0.0000   -0.0023    0.0032   -0.0000];

    if state < 4 && sim_time > 2
            
        joint_ref    = joint_references(state,:)';
        
    elseif state >= 4
        
        joint_ref    = joint_references(3,:)';
        
    end
              
end

== matlab function Robot system/controller_QP/Balancing Controller  ==
  data: tauModel output double; Sigma output double; NA output double; f_HDot output double; HessianMatrixQP1Foot output double; gradientQP1Foot output double; ConstraintsMatrixQP1Foot output double; bVectorConstraintsQp1Foot output double; HessianMatrixQP2FeetOrLegs output double; gradientQP2FeetOrLegs output double; ConstraintsMatrixQP2FeetOrLegs output double; bVectorConstraintsQp2FeetOrLegs output double; constraints input double; ROBOT_DOF_FOR_SIMULINK input double; HUMAN_DOF_FOR_SIMULINK input double; ConstraintsMatrix input double; bVectorConstraints input double; qj input double; qjDes input double; nu input double; M input double; h input double; L input double; intLw input double; w_H_l_contact input double; w_H_r_contact input double; JL input double; JR input double; dJL_nu input double; dJR_nu input double; xCoM input double; J_CoM input double; desired_x_dx_ddx_CoM input double; CMM input double; gainsPCOM input double; gainsDCOM input double; impedances input double; Reg parameter double; errorCoM output double; f_noQP output double; Gain parameter double; w_H_lArm input double; w_H_rArm input double; JLArm input double; JRArm input double; dJLArm_nu input double; dJRArm_nu input double; LArmWrench input double; RArmWrench input double; STANDUP_WITH_HUMAN_FORCE input double; MEASURED_FT input double; STANDUP_WITH_HUMAN_TORQUE input double; human_w_H_b input double; human_qj input double; human_nu_b input double; human_dqj input double; human_M input double; human_h input double; human_torques input double; human_w_H_l_contact input double; human_w_H_r_contact input double; human_JL input double; human_JR input double; human_dJL_nu input double; human_dJR_nu input double; human_w_H_lArm_contact input double; human_w_H_rArm_contact input double; human_JLArm input double; human_JRArm input double; human_dJLArm_nu input double; human_dJRArm_nu input double; correctionFromSupportForce output double; L_error output double; V output double; alpha output double; state input double; robot_torques input double; fArms output double; phri_human_feet_wrench output double; phri_robot_feet_wrench output double; correctionFromSupportTorque output double
function [tauModel, Sigma, NA, f_HDot, ...
          HessianMatrixQP1Foot, gradientQP1Foot, ConstraintsMatrixQP1Foot, bVectorConstraintsQp1Foot, ...
          HessianMatrixQP2FeetOrLegs, gradientQP2FeetOrLegs, ConstraintsMatrixQP2FeetOrLegs, bVectorConstraintsQp2FeetOrLegs, ...
          errorCoM, f_noQP, correctionFromSupportForce, L_error, V, alpha, fArms, phri_human_feet_wrench, phri_robot_feet_wrench, correctionFromSupportTorque] =  ...
              balancingControllerStandupFCN(constraints, ROBOT_DOF_FOR_SIMULINK, HUMAN_DOF_FOR_SIMULINK, ConstraintsMatrix, bVectorConstraints, ...
                                         qj, qjDes, nu, M, h, L, intLw, w_H_l_contact, w_H_r_contact, JL, JR, dJL_nu, dJR_nu, xCoM, J_CoM, desired_x_dx_ddx_CoM, CMM, ...
                                         gainsPCOM, gainsDCOM, impedances, Reg, Gain, w_H_lArm, w_H_rArm, JLArm, JRArm, dJLArm_nu, dJRArm_nu,...
                                         LArmWrench, RArmWrench, STANDUP_WITH_HUMAN_FORCE, MEASURED_FT, STANDUP_WITH_HUMAN_TORQUE, ...
                                         human_w_H_b, human_qj, human_nu_b, human_dqj, human_M, human_h, human_torques, ...
                                         human_w_H_l_contact, human_w_H_r_contact, human_JL, human_JR, human_dJL_nu, human_dJR_nu,...
                                         human_w_H_lArm_contact, human_w_H_rArm_contact, human_JLArm, human_JRArm, human_dJLArm_nu, human_dJRArm_nu,...
                                         state, robot_torques)
           
   [tauModel, Sigma, NA, f_HDot, ...
          HessianMatrixQP1Foot, gradientQP1Foot, ConstraintsMatrixQP1Foot, bVectorConstraintsQp1Foot, ...
          HessianMatrixQP2FeetOrLegs, gradientQP2FeetOrLegs, ConstraintsMatrixQP2FeetOrLegs, bVectorConstraintsQp2FeetOrLegs, ...
          errorCoM, f_noQP, correctionFromSupportForce, L_error, V, alpha, fArms, phri_human_feet_wrench, phri_robot_feet_wrench, correctionFromSupportTorque] =  ...
              balancingControllerStandup(constraints, ROBOT_DOF_FOR_SIMULINK, HUMAN_DOF_FOR_SIMULINK, ConstraintsMatrix, bVectorConstraints, ...
                                         qj, qjDes, nu, M, h, L, intLw, w_H_l_contact, w_H_r_contact, JL, JR, dJL_nu, dJR_nu, xCoM, J_CoM, desired_x_dx_ddx_CoM, CMM, ...
                                         gainsPCOM, gainsDCOM, impedances, Reg, Gain, w_H_lArm, w_H_rArm, JLArm, JRArm, dJLArm_nu, dJRArm_nu,...
                                         LArmWrench, RArmWrench, STANDUP_WITH_HUMAN_FORCE, MEASURED_FT, STANDUP_WITH_HUMAN_TORQUE, ...
                                         human_w_H_b, human_qj, human_nu_b, human_dqj, human_M, human_h, human_torques, ...
                                         human_w_H_l_contact, human_w_H_r_contact, human_JL, human_JR, human_dJL_nu, human_dJR_nu,...
                                         human_w_H_lArm_contact, human_w_H_rArm_contact, human_JLArm, human_JRArm, human_dJLArm_nu, human_dJRArm_nu,...
                                         state, robot_torques);
end

== matlab function Robot system/emergency stop: joint limits/MATLAB Function ==
  data: umin input double; umax input double; u input double; inRange output double; tol input double
function inRange = checkRangeFCN(umin, umax, u, tol)

    inRange = checkRange(umin, umax, u, tol);
end

== matlab function Robot system/controller_QP/Compute angular momentum integral/References for H ==
  data: qjErr input double; JL input double; JR input double; nu_b_equivalent output double; Reg parameter double; activeFeetConstraints input double
function nu_b_equivalent = generateReferencesForH_FCN(qjErr, JL, JR, Reg, activeFeetConstraints)

    if activeFeetConstraints(1) == 1
    
        pinvJb          = (JL(:,1:6)'*JL(:,1:6) + Reg.pinvDamp_nu_b*eye(6))\JL(:,1:6)';
        nu_b_equivalent = -pinvJb*JL(:,7:end)*qjErr;
    else
    
        pinvJb          = (JR(:,1:6)'*JR(:,1:6) + Reg.pinvDamp_nu_b*eye(6))\JR(:,1:6)';
        nu_b_equivalent = -pinvJb*JR(:,7:end)*qjErr;
    end
end

== matlab function Robot system/Robot State and References/State Machine Standup/Visualise extrnal wrenches/Compute current threshold ==
  data: thresholdContactLeftHand output double; thresholdContactRightHand output double; state input double; thresholdContactLeftFoot output double; thresholdContactRightFoot output double; Sm parameter double
function [thresholdContactLeftHand,thresholdContactRightHand, ...
          thresholdContactLeftFoot,thresholdContactRightFoot] = currentThreshold(state,Sm)

    thresholdContactLeftHand  = Sm.wrench_thresholdContactLHand(state);
    thresholdContactRightHand = Sm.wrench_thresholdContactRHand(state);
    thresholdContactLeftFoot  = Sm.wrench_thresholdContactLFoot(state);
    thresholdContactRightFoot = Sm.wrench_thresholdContactRFoot(state);
end
